simulink model "State_Space_Simulation"  (R2019a)
settings: Solver=VariableStepAuto  StartTime=0.0  StopTime=2  RelTol=1e-3
values from neighbouring files (symbols this model uses):
  A = 1/5    (= 0.2)    [Pendulum_SS_Init.m]    (also in Pendulum_State_Space.m = [0, 1; -a, -b])
  B = [0, b]'    [Pendulum_State_Space.m]
  C = eye(2)    [Pendulum_State_Space.m]
  G = [1, 0]'    [Pendulum_State_Space.m]
  K = place(A,B, [-10, -20])    [Pendulum_State_Space.m]
undefined symbols (not defined in the file or in its folder): Ki
settings Model: Creator=QuarcUser  LastModifiedBy=QuarcUser

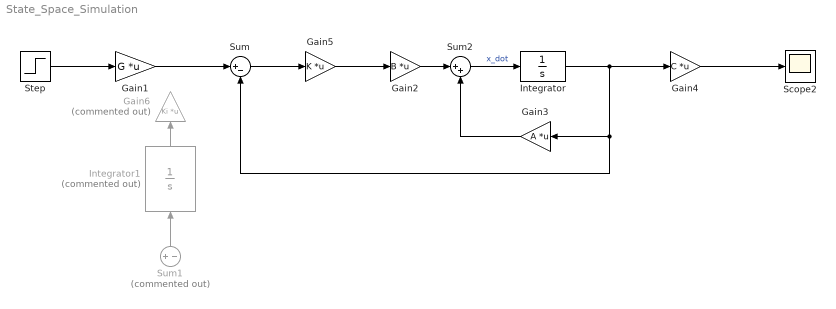
== system State_Space_Simulation ==
  Gain1 : Gain  Gain=G  Multiplication=Matrix(K*u)
  Gain2 : Gain  Gain=B  Multiplication=Matrix(K*u)
  Gain3 : Gain  Gain=A  Multiplication=Matrix(K*u)
  Gain4 : Gain  Gain=C  Multiplication=Matrix(K*u)
  Gain5 : Gain  Gain=K  Multiplication=Matrix(K*u)
  Gain6 : Gain  Commented=on  Gain=Ki  Multiplication=Matrix(K*u)
  Integrator : Integrator  InitialCondition=[0;0]
  Integrator1 : Integrator  Commented=on  InitialCondition=[0;0]
  Scope2 : Scope
  Step : Step  SampleTime=.002
  Sum : Sum  Inputs=|+-
  Sum1 : Sum  Commented=on  Inputs=+-
  Sum2 : Sum  Inputs=|++
  wires:
  Step/1 -> Gain1/1
  Gain1/1 -> Sum/1
  Sum/1 -> Gain5/1
  Gain2/1 -> Sum2/1
  Sum2/1 -> Integrator/1  "x_dot"
  Gain3/1 -> Sum2/2
  Sum1/1 -> Integrator1/1
  Gain4/1 -> Scope2/1
  Integrator1/1 -> Gain6/1
  Integrator/1 -> Gain3/1, Sum/2, Gain4/1
  Gain5/1 -> Gain2/1
